simulink model "pidcontrol"  (Simulink 7.1)
settings: Solver=ode45  StartTime=0.0  StopTime=10.0  RelTol=1e-3
values from neighbouring files (symbols this model uses):
  g = 9.81    [pid_parameters.m]    (also in sample_file.m)
  I = 0.0068    [pid_parameters.m]    (also in sample_file.m = 0.05)
  Kd = -5    [pid_parameters.m]
  Ki = -5    [pid_parameters.m]
  Kp = -20    [pid_parameters.m]
  l = 0.4    [pid_parameters.m]    (also in sample_file.m = 0.3)
  M = 0.6    [pid_parameters.m]    (also in sample_file.m = 0.5)
  m = 0.09    [pid_parameters.m]    (also in sample_file.m = 0.2)
settings Model: Creator=minakata  LastModifiedBy=minakata

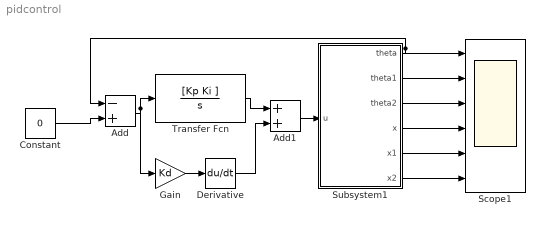
== system pidcontrol ==
  Add : Sum  Inputs=-+  OutDataType=sfix(16)  OutScaling=2^-10
  Add1 : Sum  OutDataType=sfix(16)  OutScaling=2^-10
  Constant : Constant  Value=0  OutDataType=sfix(16)  OutScaling=2^0
  Derivative : Derivative
  Gain : Gain  Gain=Kd  ParameterDataType=sfix(16)  ParameterScaling=2^0  OutDataType=sfix(16)  OutScaling=2^0
  Scope1 : Scope  NumInputPorts=6
      settings: TimeRange=10  YMin=-10~-10~-50~0~-10~-20  YMax=20~10~50~60~20~20
  Subsystem1 : Subsystem
  Transfer Fcn : TransferFcn  Numerator=[Kp Ki ]  Denominator=[ 1 0]
  wires:
  Constant/1 -> Add/2
  Subsystem1/1(theta) -> Add/1, Scope1/1
  Add/1 -> Transfer Fcn/1, Gain/1
  Subsystem1/2(theta1) -> Scope1/2
  Subsystem1/3(theta2) -> Scope1/3
  Subsystem1/4(x) -> Scope1/4
  Subsystem1/5(x1) -> Scope1/5
  Subsystem1/6(x2) -> Scope1/6
  Gain/1 -> Derivative/1
  Add1/1 -> Subsystem1/1(u)
  Transfer Fcn/1 -> Add1/1
  Derivative/1 -> Add1/2

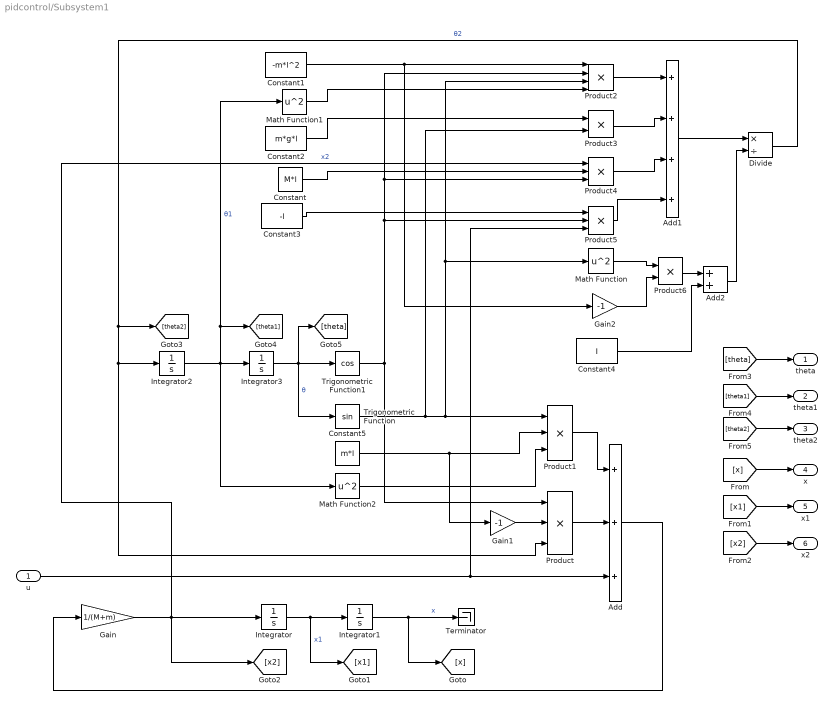
== system pidcontrol/Subsystem1 ==
  u : Inport  OutDataType=sfix(16)  OutScaling=2^0
  Add : Sum  Inputs=+++  OutDataType=sfix(16)  OutScaling=2^-10
  Add1 : Sum  Inputs=++++  OutDataType=sfix(16)  OutScaling=2^-10
  Add2 : Sum  OutDataType=sfix(16)  OutScaling=2^-10
  Constant : Constant  Value=M*l  OutDataType=sfix(16)  OutScaling=2^0
  Constant1 : Constant  Value=-m*l^2  OutDataType=sfix(16)  OutScaling=2^0
  Constant2 : Constant  Value=m*g*l  OutDataType=sfix(16)  OutScaling=2^0
  Constant3 : Constant  Value=-l  OutDataType=sfix(16)  OutScaling=2^0
  Constant4 : Constant  Value=I  OutDataType=sfix(16)  OutScaling=2^0
  Constant5 : Constant  Value=m*l  OutDataType=sfix(16)  OutScaling=2^0
  Divide : Product  Inputs=*/  OutDataType=sfix(16)  OutScaling=2^-10
  Gain : Gain  Gain=1/(M+m)  ParameterDataType=sfix(16)  ParameterScaling=2^0  OutDataType=sfix(16)  OutScaling=2^0
  Gain1 : Gain  Gain=-1  ParameterDataType=sfix(16)  ParameterScaling=2^0  OutDataType=sfix(16)  OutScaling=2^0
  Gain2 : Gain  Gain=-1  ParameterDataType=sfix(16)  ParameterScaling=2^0  OutDataType=sfix(16)  OutScaling=2^0
  Integrator : Integrator
  Integrator1 : Integrator
  Integrator2 : Integrator
  Integrator3 : Integrator  InitialCondition=0.1
  Math Function : Math  Operator=square  OutDataType=sfix(16)  OutScaling=2^0  SaturateOnIntegerOverflow=on
  Math Function1 : Math  Operator=square  OutDataType=sfix(16)  OutScaling=2^0  SaturateOnIntegerOverflow=on
  Math Function2 : Math  Operator=square  OutDataType=sfix(16)  OutScaling=2^0  SaturateOnIntegerOverflow=on
  Product{,1,4..5} (4 alike) : Product  Inputs=3  OutDataType=sfix(16)  OutScaling=2^0  RndMeth=Zero
  Product2 : Product  Inputs=4  OutDataType=sfix(16)  OutScaling=2^0  RndMeth=Zero
  Product3 : Product  OutDataType=sfix(16)  OutScaling=2^0  RndMeth=Zero
  Product6 : Product  OutDataType=sfix(16)  OutScaling=2^0  RndMeth=Zero
  Terminator : Terminator
  Trigonometric Function : Trigonometry
  Trigonometric Function1 : Trigonometry  Operator=cos
  theta : Outport  OutDataType=sfix(16)  OutScaling=2^0
  theta1 : Outport  Port=2  OutDataType=sfix(16)  OutScaling=2^0
  theta2 : Outport  Port=3  OutDataType=sfix(16)  OutScaling=2^0
  x : Outport  Port=4  OutDataType=sfix(16)  OutScaling=2^0
  x1 : Outport  Port=5  OutDataType=sfix(16)  OutScaling=2^0
  x2 : Outport  Port=6  OutDataType=sfix(16)  OutScaling=2^0
  wires:
  [x] -> x/1
  [x1] -> x1/1
  [x2] -> x2/1
  [theta] -> theta/1
  [theta1] -> theta1/1
  [theta2] -> theta2/1
  Integrator1/1 -> Terminator/1, [x]  "x"
  Add/1 -> Gain/1
  u/1 -> Product5/3, Add/3
  Add1/1 -> Divide/1
  Add2/1 -> Divide/2
  Constant4/1 -> Add2/2
  Product6/1 -> Add2/1
  Math Function/1 -> Product6/1
  Product5/1 -> Add1/4
  Product4/1 -> Add1/3
  Product3/1 -> Add1/2
  Product2/1 -> Add1/1
  Constant3/1 -> Product5/1
  Constant2/1 -> Product3/1
  Constant1/1 -> Product2/1, Gain2/1
  Product1/1 -> Add/1
  Trigonometric Function1/1 -> Product2/2, Product4/3, Product5/2, Product/1
  Product/1 -> Add/2
  Constant/1 -> Product4/2
  Trigonometric Function/1 -> Product3/2, Product2/3, Math Function/1, Product1/1
  Integrator3/1 -> Trigonometric Function/1, Trigonometric Function1/1, [theta]  "θ"
  Integrator2/1 -> [theta1], Math Function1/1, Integrator3/1, Math Function2/1  "θ1"
  Divide/1 -> Integrator2/1, Product/3, [theta2]  "θ2"
  Integrator/1 -> Integrator1/1, [x1]  "x1"
  Gain/1 -> Product4/1, Integrator/1, [x2]  "x2"
  Math Function1/1 -> Product2/4
  Gain2/1 -> Product6/2
  Gain1/1 -> Product/2
  Math Function2/1 -> Product1/3
  Constant5/1 -> Product1/2, Gain1/1
